simulink model "q1model"  (R2023b)
settings: Solver=ode23tb  StartTime=0.0  StopTime=8  MaxStep=1e-3  RelTol=1e-4  AbsTol=1e-4
values from neighbouring files (symbols this model uses):
  J = 0.00022    [circuit_params.mat]    (also in parameters.m)
  lambdam = 0.0215    [circuit_params.mat]    (also in parameters.m)
  Lss = 0.000375    [circuit_params.mat]    (also in parameters.m)
  p = 8    [circuit_params.mat]    (also in parameters.m)
  rs = 0.25    [circuit_params.mat]    (also in parameters.m)
  Tfirc = 0.12    [circuit_params.mat]    (also in parameters.m)
  vdc = 45    [circuit_params.mat]    (also in parameters.m)
libraries: matrix_library x1
settings Model: Creator=jianghaoyuan  LastModifiedBy=10099
settings RTWCC: GPUComputeCapability=5.0

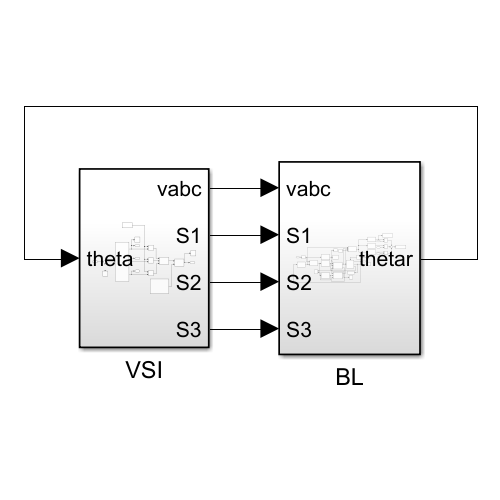
[thumbnail: Simulink's stored preview of the top-level diagram]
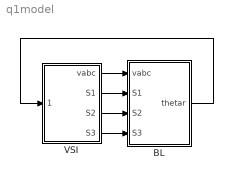
== system q1model ==
  BL : Subsystem
  VSI : Subsystem
  wires:
  VSI/1(vabc) -> BL/1(vabc)
  BL/1(thetar) -> VSI/1(theta)
  VSI/2(S1) -> BL/2(S1)
  VSI/3(S2) -> BL/3(S2)
  VSI/4(S3) -> BL/4(S3)

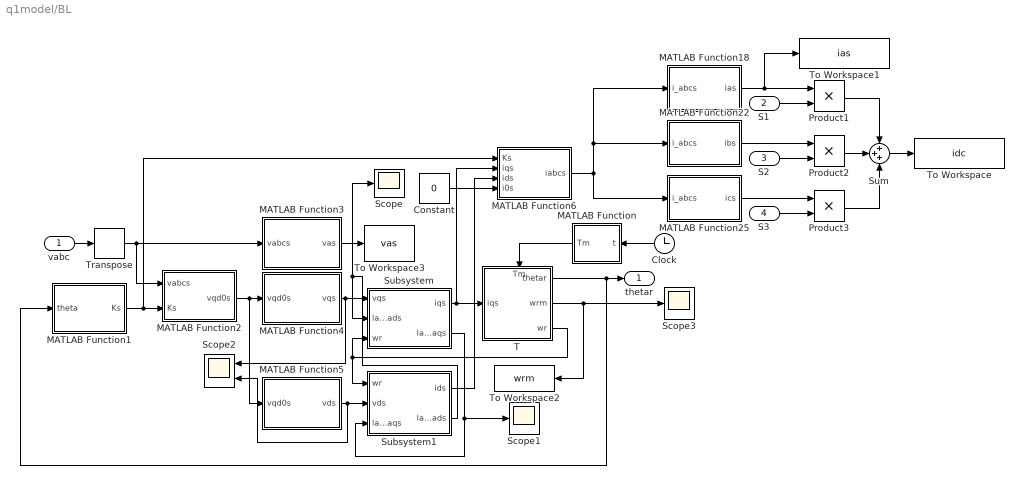
== system q1model/BL ==
  vabc : Inport
  S1 : Inport  Port=2
  S2 : Inport  Port=3
  S3 : Inport  Port=4
  Clock : Clock
      settings: Decimation=2
  Constant : Constant  Value=0
  MATLAB Function : MATLAB Function  TreatAsAtomicUnit=on
  MATLAB Function1 : MATLAB Function  TreatAsAtomicUnit=on
  MATLAB Function18 : MATLAB Function  TreatAsAtomicUnit=on
  MATLAB Function2 : MATLAB Function  TreatAsAtomicUnit=on
  MATLAB Function22 : MATLAB Function  TreatAsAtomicUnit=on
  MATLAB Function25 : MATLAB Function  TreatAsAtomicUnit=on
  MATLAB Function3 : MATLAB Function  TreatAsAtomicUnit=on
  MATLAB Function4 : MATLAB Function  TreatAsAtomicUnit=on
  MATLAB Function5 : MATLAB Function  TreatAsAtomicUnit=on
  MATLAB Function6 : MATLAB Function  TreatAsAtomicUnit=on
  Product1 : Product
  Product2 : Product
  Product3 : Product
  Scope : Scope
  Scope1 : Scope
  Scope2 : Scope  NumInputPorts=2
  Scope3 : Scope
  Subsystem : Subsystem
  Subsystem1 : Subsystem
  Sum : Sum  Inputs=+++
  T : Subsystem
      settings: PortSchema="{\"entries\":[{\"content\":{\"sides\":[{\"content\":{\"connectorIds\":[\"In1\"]},\"type\":\"ConnectorPlacement.EquallySpacedRectSide\",\"uuid\":\"81cf2644-7574-48ea-89e0-b270508e1d33\"},{\"content\":{\"connectorIds\":[\"Out1\",\"Out2\",\"Out3\"],\"side\":\"RIGHT\"},\"type\":\"ConnectorPlacement.EquallySpacedRectSide\",\"uuid\":\"07c3c316-7b78-417d-8688-d2de0bc324fc\"},{\"content\":{\"connectorIds\":[\"In2\"],\"side\":\"TOP\"},\"type\":\"ConnectorPlacement.EquallySpacedRectSide\",\"uuid\":\"d73af36a-209b-49ab-900f-ad4819e2f625\"}]},\"type\":\"ConnectorPlacement.EquallySpacedConnector\",\"uuid\":\"0682574c-ecfc-4979-9c95-a0d0804321ad\"}],\"packageUris\":[\"http://schema.mathworks.com/mf0/Connector/R2020b\"],\"version\":\"1.0\"}"
  To Workspace : ToWorkspace  VariableName=idc  SaveFormat=Timeseries  SampleTime=-1
  To Workspace1 : ToWorkspace  VariableName=ias  SaveFormat=Timeseries  SampleTime=-1
  To Workspace2 : ToWorkspace  VariableName=wrm  SaveFormat=Timeseries  SampleTime=-1
  To Workspace3 : ToWorkspace  VariableName=vas  SaveFormat=Timeseries  SampleTime=-1
  Transpose : matrix_library/Transpose
  thetar : Outport
  wires:
  MATLAB Function2/1(vqd0s) -> MATLAB Function5/1(vqd0s), MATLAB Function4/1(vqd0s)
  vabc/1 -> Transpose/1
  MATLAB Function4/1(vqs) -> Scope2/1, Subsystem/1(vqs)
  Transpose/1 -> MATLAB Function2/1(vabcs), MATLAB Function3/1(vabcs)
  T/1(thetar) -> MATLAB Function1/1(theta), thetar/1
  Subsystem/1(iqs) -> MATLAB Function6/2(iqs), T/1(iqs)
  Clock/1 -> MATLAB Function/1(t)
  MATLAB Function/1(Tm) -> T/2(Tm)
  MATLAB Function1/1(Ks) -> MATLAB Function6/1(Ks), MATLAB Function2/2(Ks)
  T/2(wrm) -> Scope3/1, To Workspace2/1
  MATLAB Function3/1(vas) -> To Workspace3/1
  T/3(wr) -> Subsystem/3(wr), Subsystem1/1(wr)
  MATLAB Function5/1(vds) -> Subsystem1/2(vds), Scope2/2
  Subsystem/2(lambdaqs) -> Subsystem1/3(lamdaqs), Scope1/1
  Subsystem1/2(lambdads) -> Subsystem/2(lamdads), Scope/1
  MATLAB Function22/1(ibs) -> Product2/1
  MATLAB Function18/1(ias) -> To Workspace1/1, Product1/1
  S2/1 -> Product2/2
  S3/1 -> Product3/2
  MATLAB Function25/1(ics) -> Product3/1
  S1/1 -> Product1/2
  MATLAB Function6/1(iabcs) -> MATLAB Function18/1(i_abcs), MATLAB Function22/1(i_abcs), MATLAB Function25/1(i_abcs)
  Subsystem1/1(ids) -> MATLAB Function6/3(ids)
  Constant/1 -> MATLAB Function6/4(i0s)
  Product2/1 -> Sum/2
  Product1/1 -> Sum/1
  Product3/1 -> Sum/3
  Sum/1 -> To Workspace/1

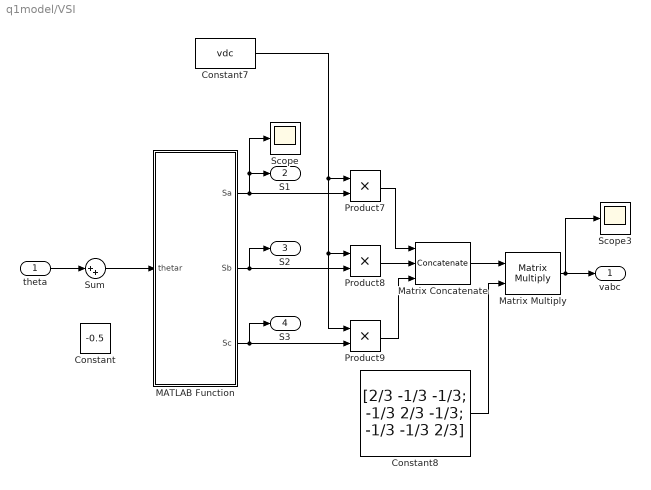
== system q1model/VSI ==
  theta : Inport
  Constant : Constant  Value=-0.5
  Constant7 : Constant  Value=vdc
  Constant8 : Constant  Value=[2/3 -1/3 -1/3; -1/3 2/3 -1/3; -1/3 -1/3 2/3]
  MATLAB Function : MATLAB Function  TreatAsAtomicUnit=on
  Matrix Concatenate : Concatenate  NumInputs=3  Mode=Multidimensional array  ConcatenateDimension=2
  Matrix Multiply : Product  Multiplication=Matrix(*)
  Product7 : Product
  Product8 : Product
  Product9 : Product
  Scope : Scope
  Scope3 : Scope
  Sum : Sum  Inputs=|++
  vabc : Outport
  S1 : Outport  Port=2
  S2 : Outport  Port=3
  S3 : Outport  Port=4
  wires:
  Product7/1 -> Matrix Concatenate/1
  Matrix Multiply/1 -> vabc/1, Scope3/1
  Constant8/1 -> Matrix Multiply/2
  Product9/1 -> Matrix Concatenate/3
  Product8/1 -> Matrix Concatenate/2
  Matrix Concatenate/1 -> Matrix Multiply/1
  MATLAB Function/1(Sa) -> Scope/1, S1/1, Product7/2
  MATLAB Function/2(Sb) -> S2/1, Product8/2
  MATLAB Function/3(Sc) -> S3/1, Product9/2
  theta/1 -> Sum/1
  Sum/1 -> MATLAB Function/1(thetar)
  Constant7/1 -> Product9/1, Product8/1, Product7/1

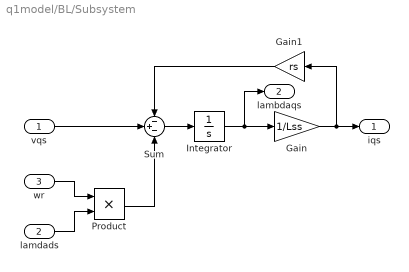
== system q1model/BL/Subsystem ==
  vqs : Inport
  lamdads : Inport  Port=2
  wr : Inport  Port=3
  Gain : Gain  Gain=1/Lss
  Gain1 : Gain  Gain=rs
  Integrator : Integrator
  Product : Product
  Sum : Sum  Inputs=-+-
  iqs : Outport
  lambdaqs : Outport  Port=2
  wires:
  wr/1 -> Product/1
  lamdads/1 -> Product/2
  vqs/1 -> Sum/2
  Product/1 -> Sum/3
  Sum/1 -> Integrator/1
  Gain/1 -> Gain1/1, iqs/1
  Gain1/1 -> Sum/1
  Integrator/1 -> lambdaqs/1, Gain/1

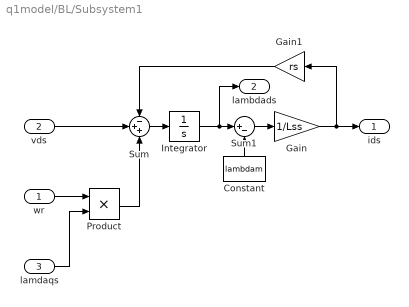
== system q1model/BL/Subsystem1 ==
  wr : Inport
  vds : Inport  Port=2
  lamdaqs : Inport  Port=3
  Constant : Constant  Value=lambdam
  Gain : Gain  Gain=1/Lss
  Gain1 : Gain  Gain=rs
  Integrator : Integrator
  Product : Product
  Sum : Sum  Inputs=-++
  Sum1 : Sum  Inputs=|+-
  ids : Outport
  lambdads : Outport  Port=2
  wires:
  wr/1 -> Product/1
  lamdaqs/1 -> Product/2
  vds/1 -> Sum/2
  Product/1 -> Sum/3
  Sum/1 -> Integrator/1
  Gain/1 -> Gain1/1, ids/1
  Gain1/1 -> Sum/1
  Sum1/1 -> Gain/1
  Integrator/1 -> lambdads/1, Sum1/1
  Constant/1 -> Sum1/2

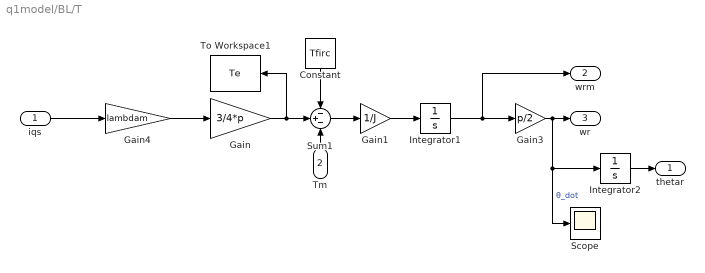
== system q1model/BL/T ==
  iqs : Inport
  Tm : Inport  Port=2
  Constant : Constant  Value=Tfirc
  Gain : Gain  Gain=3/4*p
  Gain1 : Gain  Gain=1/J
  Gain3 : Gain  Gain=p/2
  Gain4 : Gain  Gain=lambdam
  Integrator1 : Integrator
  Integrator2 : Integrator
  Scope : Scope
  Sum1 : Sum  Inputs=-+-
  To Workspace1 : ToWorkspace  VariableName=Te  SaveFormat=Timeseries  SampleTime=-1
  thetar : Outport
  wrm : Outport  Port=2
  wr : Outport  Port=3
  wires:
  Gain/1 -> To Workspace1/1, Sum1/2
  Gain1/1 -> Integrator1/1
  Integrator1/1 -> wrm/1, Gain3/1
  Gain3/1 -> Scope/1, Integrator2/1, wr/1  "θ_dot"
  Integrator2/1 -> thetar/1
  Tm/1 -> Sum1/3
  Sum1/1 -> Gain1/1
  Constant/1 -> Sum1/1
  iqs/1 -> Gain4/1
  Gain4/1 -> Gain/1

== matlab function q1model/BL/MATLAB Function1 ==
  data: theta input; Ks output
function Ks = Ks(theta)

Ks = 2/3*[cos(theta), cos(theta-2/3*pi), cos(theta+2/3*pi);
          sin(theta), sin(theta-2/3*pi), sin(theta+2/3*pi);
          1/2, 1/2, 1/2];

== matlab function q1model/VSI/MATLAB Function ==
  data: thetar input; Sa output; Sb output; Sc output
function [Sa, Sb, Sc] = fcn(thetar)
    thetar = wrapTo360(rad2deg(thetar));
    if thetar > 30 && thetar <= 90
        Sa = 1;
        Sb = 1;
        Sc = 0;
    elseif thetar > 90 && thetar <= 150
        Sa = 0;
        Sb = 1;
        Sc = 0;
    elseif thetar > 150 && thetar <= 210
        Sa = 0;
        Sb = 1;
        Sc = 1;
    elseif thetar > 210 && thetar <= 270
        Sa = 0;
        Sb = 0;
        Sc = 1;
    elseif thetar > 270 && thetar <= 330
        Sa = 1;
        Sb = 0;
        Sc = 1;
    else
        Sa = 1;
        Sb = 0;
        Sc = 0;
    end
end

== matlab function q1model/BL/MATLAB Function2 ==
  data: vabcs input; Ks input; vqd0s output
function vqd0s = fcn(vabcs, Ks)

vqd0s = Ks*vabcs;

== matlab function q1model/BL/MATLAB Function ==
  data: t input; Tm output
function Tm = fcn(t)
if t<1
    Tm = 0;
else
    Tm = 1.5;
end

== matlab function q1model/BL/MATLAB Function4 ==
  data: vqs output; vqd0s input
function vqs= vqs(vqd0s)

vqs = vqd0s(1);

== matlab function q1model/BL/MATLAB Function3 ==
  data: vas output; vabcs input
function vas= vas(vabcs)

vas = vabcs(1);

== matlab function q1model/BL/MATLAB Function5 ==
  data: vds output; vqd0s input
function vds= vds(vqd0s)

vds = vqd0s(2);

== matlab function q1model/BL/MATLAB Function6 ==
  data: Ks input; iqs input; ids input; iabcs output; i0s input
function iabcs = iabcs(Ks, iqs, ids, i0s)
    
    iqd0s = zeros(3,1);
    iqd0s(1) = iqs;
    iqd0s(2) = ids;
    iqd0s(3) = i0s;
    iabcs = inv(Ks)*iqd0s;

== matlab function q1model/BL/MATLAB Function18 ==
  data: i_abcs input; ias output
function ias = ias(i_abcs)

ias = i_abcs(1);

== matlab function q1model/BL/MATLAB Function22 ==
  data: i_abcs input; ibs output
function ibs = ibs(i_abcs)

ibs = i_abcs(2);

== matlab function q1model/BL/MATLAB Function25 ==
  data: i_abcs input; ics output
function ics = ics(i_abcs)

ics = i_abcs(3);
